simulink model "ex3"  (R2016a)
settings: Solver=VariableStepAuto  StartTime=0.0  StopTime=inf  RelTol=1e-3
settings Model: Creator=Utilizator  LastModifiedBy=Utilizator

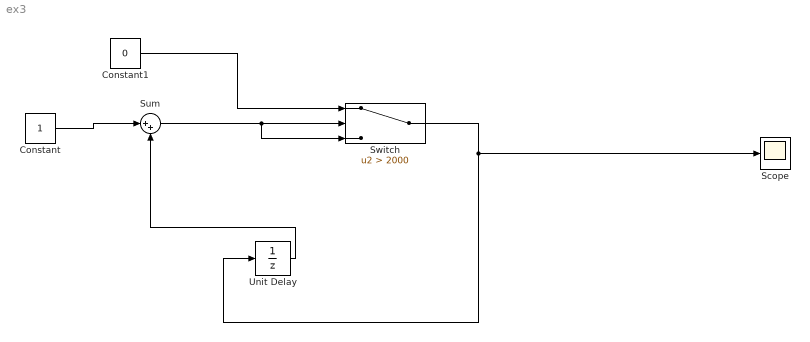
== system ex3 ==
  Constant : Constant
  Constant1 : Constant  Value=0
  Scope : Scope
  Sum : Sum  Inputs=|++
  Switch : Switch  Criteria=u2 > Threshold  Threshold=2000
  Unit Delay : UnitDelay  SampleTime=1000
  wires:
  Constant/1 -> Sum/1
  Sum/1 -> Switch/3, Switch/2
  Constant1/1 -> Switch/1
  Switch/1 -> Unit Delay/1, Scope/1
  Unit Delay/1 -> Sum/2
